simulink model "tests_and_trash"  (R2021b)
settings: Solver=VariableStepAuto  StartTime=0.0  StopTime=TMax  FixedStep=dtMax  MaxStep=dtMax  RelTol=1e-5
undefined symbols (not defined in the file or in its folder): airgap, intensity, pod
libraries: shared6dof x1
settings Model: Creator=Ferran  LastModifiedBy=Ferran
settings SolverCC: MaxConsecutiveMinStep=3

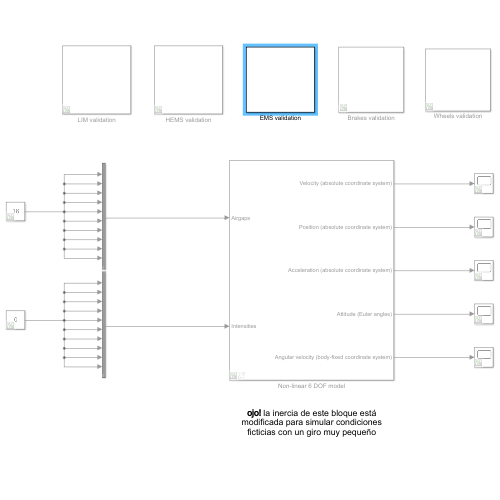
[thumbnail: Simulink's stored preview of the top-level diagram]
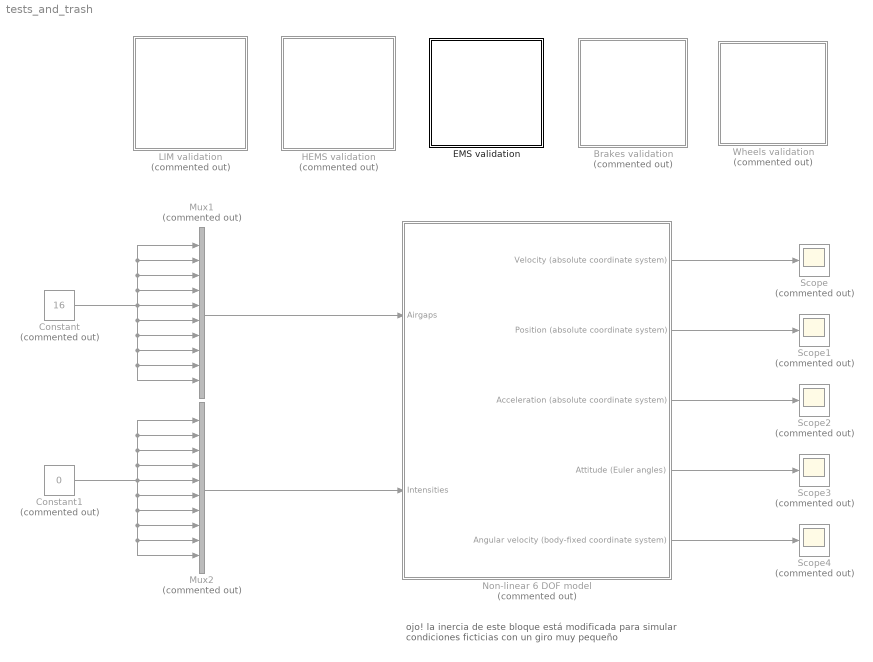
== system tests_and_trash ==
  note: ojo! la inercia de este bloque está modificada para simular condiciones ficticias con un giro muy pequeño
  Brakes validation : Subsystem  Commented=on
  Constant : Constant  Commented=on  Value=16
  Constant1 : Constant  Commented=on  Value=0
  EMS validation : Subsystem
  HEMS validation : Subsystem  Commented=on
  LIM validation : Subsystem  Commented=on
  Mux1 : Mux  Commented=on  Inputs=10
  Mux2 : Mux  Commented=on  Inputs=10
  Non-linear 6 DOF model : Subsystem  Commented=on  AncestorBlock=libH7/Non-linear 6 DOF model
  Scope{,1..4} (5 alike) : Scope  Commented=on
  Wheels validation : Subsystem  Commented=on
  wires:
  Mux2/1 -> Non-linear 6 DOF model/2(Intensities)
  Constant1/1 -> Mux2/2, Mux2/1, Mux2/3, Mux2/4, Mux2/9, Mux2/10, Mux2/8, Mux2/7, Mux2/6, Mux2/5
  Mux1/1 -> Non-linear 6 DOF model/1(Airgaps)
  Non-linear 6 DOF model/1(Velocity (absolute coordinate system)) -> Scope/1
  Non-linear 6 DOF model/2(Position (absolute coordinate system)) -> Scope1/1
  Non-linear 6 DOF model/3(Acceleration (absolute coordinate system)) -> Scope2/1
  Non-linear 6 DOF model/4(Attitude (Euler angles)) -> Scope3/1
  Non-linear 6 DOF model/5(Angular velocity (body-fixed coordinate system)) -> Scope4/1
  Constant/1 -> Mux1/2, Mux1/1, Mux1/3, Mux1/4, Mux1/9, Mux1/10, Mux1/8, Mux1/7, Mux1/6, Mux1/5

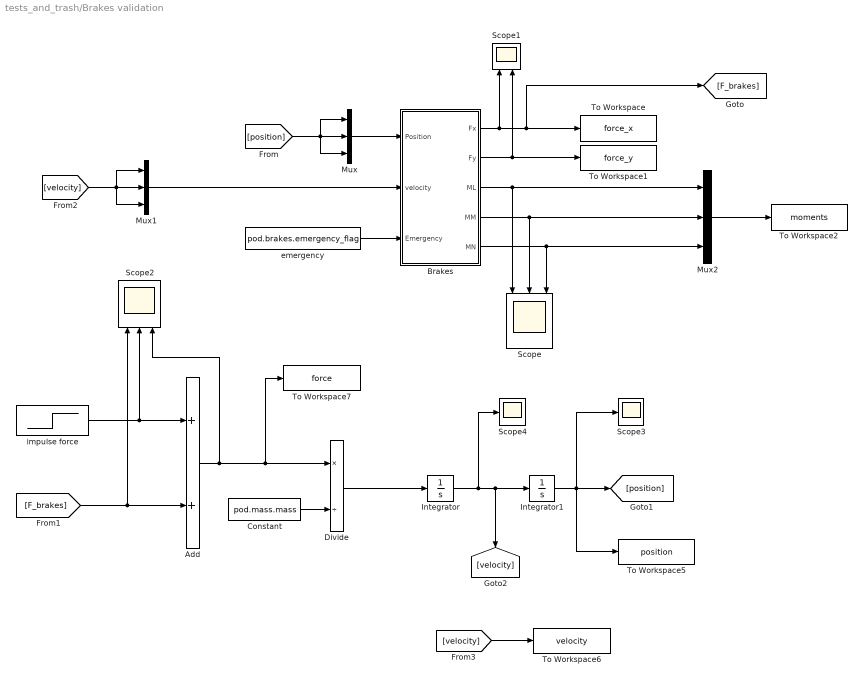
== system tests_and_trash/Brakes validation ==
  Add : Sum  Inputs=2
  Brakes : Subsystem
  Constant : Constant  Value=pod.mass.mass
  Divide : Product  Inputs=*/
  Integrator : Integrator
  Integrator1 : Integrator
  Mux : Mux  Inputs=3
  Mux1 : Mux  Inputs=3
  Mux2 : Mux  Inputs=3
  Scope : Scope  NumInputPorts=3
  Scope1 : Scope  NumInputPorts=2
  Scope2 : Scope  NumInputPorts=3
  Scope3 : Scope
  Scope4 : Scope
  To Workspace : ToWorkspace  VariableName=force_x  SaveFormat=Timeseries  SampleTime=-1
  To Workspace1 : ToWorkspace  VariableName=force_y  SaveFormat=Timeseries  SampleTime=-1
  To Workspace2 : ToWorkspace  VariableName=moments  SaveFormat=Timeseries  SampleTime=-1
  To Workspace5 : ToWorkspace  VariableName=position  SaveFormat=Timeseries  SampleTime=-1
  To Workspace6 : ToWorkspace  VariableName=velocity  SaveFormat=Timeseries  SampleTime=-1
  To Workspace7 : ToWorkspace  VariableName=force  SaveFormat=Timeseries  SampleTime=-1
  emergency : Constant  Value=pod.brakes.emergency_flag
  impulse force : Step  Before=1000  After=0  SampleTime=0
  wires:
  Brakes/1(Fx) -> Scope1/1, To Workspace/1, [F_brakes]
  Brakes/3(ML) -> Scope/1, Mux2/1
  Brakes/2(Fy) -> Scope1/2, To Workspace1/1
  Brakes/5(MN) -> Mux2/3, Scope/3
  emergency/1 -> Brakes/3(Emergency)
  Brakes/4(MM) -> Scope/2, Mux2/2
  impulse force/1 -> Add/1, Scope2/2
  Integrator/1 -> Scope4/1, Integrator1/1, [velocity]
  [F_brakes] -> Add/2, Scope2/1
  Add/1 -> To Workspace7/1, Divide/1, Scope2/3
  Constant/1 -> Divide/2
  Divide/1 -> Integrator/1
  Integrator1/1 -> To Workspace5/1, Scope3/1, [position]
  [position] -> Mux/3, Mux/1, Mux/2
  Mux/1 -> Brakes/1(Position)
  Mux1/1 -> Brakes/2(velocity)
  [velocity] -> Mux1/3, Mux1/1, Mux1/2
  [velocity] -> To Workspace6/1
  Mux2/1 -> To Workspace2/1

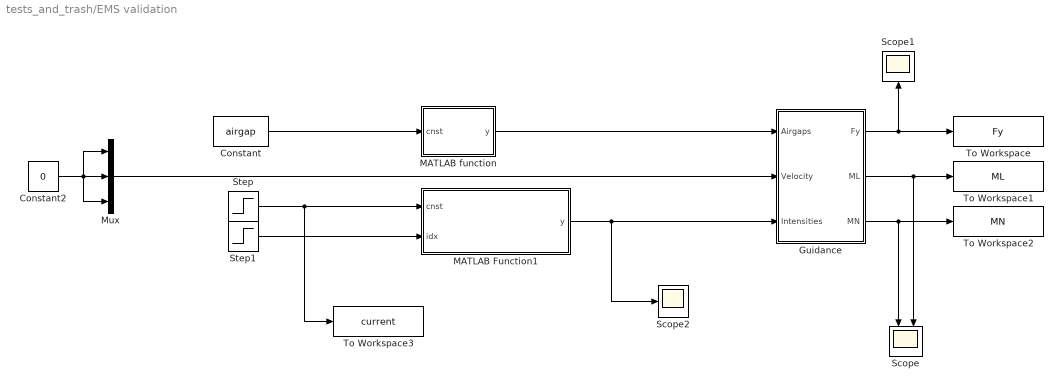
== system tests_and_trash/EMS validation ==
  Constant : Constant  Value=airgap
  Constant2 : Constant  Value=0
  Guidance : Subsystem
  MATLAB Function1 : MATLAB Function  TreatAsAtomicUnit=on
  MATLAB function : MATLAB Function  TreatAsAtomicUnit=on
  Mux : Mux  Inputs=3
  Scope : Scope  NumInputPorts=2
  Scope1 : Scope
  Scope2 : Scope
  Step : Step  Time=3  Before=intensity  After=intensity + 10  SampleTime=0
  Step1 : Step  Time=10  Before=7  After=7  SampleTime=0
  To Workspace : ToWorkspace  VariableName=Fy  SaveFormat=Timeseries  SampleTime=-1
  To Workspace1 : ToWorkspace  VariableName=ML  SaveFormat=Timeseries  SampleTime=-1
  To Workspace2 : ToWorkspace  VariableName=MN  SaveFormat=Timeseries  SampleTime=-1
  To Workspace3 : ToWorkspace  VariableName=current  SaveFormat=Timeseries  SampleTime=-1
  wires:
  Mux/1 -> Guidance/2(Velocity)
  Step/1 -> To Workspace3/1, MATLAB Function1/1(cnst)
  MATLAB function/1(y) -> Guidance/1(Airgaps)
  Constant/1 -> MATLAB function/1(cnst)
  Constant2/1 -> Mux/2, Mux/1, Mux/3
  Step1/1 -> MATLAB Function1/2(idx)
  Guidance/1(Fy) -> To Workspace/1, Scope1/1
  MATLAB Function1/1(y) -> Scope2/1, Guidance/3(Intensities)
  Guidance/2(ML) -> Scope/2, To Workspace1/1
  Guidance/3(MN) -> Scope/1, To Workspace2/1

== system tests_and_trash/HEMS validation ==
  Constant : Constant  Value=airgap
  Constant1 : Constant  Value=intensity
  Constant2 : Constant  Value=5
  Levitation : Subsystem
  MATLAB Function1 : MATLAB Function  TreatAsAtomicUnit=on
  MATLAB unction3 : MATLAB Function  TreatAsAtomicUnit=on
  Mux : Mux  Inputs=3
  Scope : Scope  NumInputPorts=2
  Scope1 : Scope  NumInputPorts=2
  Scope2 : Scope
  To Workspace : ToWorkspace  VariableName=Fx  SaveFormat=Timeseries  SampleTime=-1
  To Workspace1 : ToWorkspace  VariableName=Fz  SaveFormat=Timeseries  SampleTime=-1
  To Workspace2 : ToWorkspace  VariableName=ML  SaveFormat=Timeseries  SampleTime=-1
  To Workspace3 : ToWorkspace  VariableName=MM  SaveFormat=Timeseries  SampleTime=-1
  wires:
  Constant/1 -> MATLAB unction3/1(cnst)
  MATLAB unction3/1(y) -> Levitation/1(Airgaps)
  Constant1/1 -> MATLAB Function1/1(cnst)
  MATLAB Function1/1(y) -> Scope2/1, Levitation/3(Intensities)
  Mux/1 -> Levitation/2(Velocity)
  Levitation/1(Fx) -> Scope/2, To Workspace/1
  Levitation/2(Fz) -> Scope/1, To Workspace1/1
  Levitation/3(ML) -> To Workspace2/1, Scope1/2
  Levitation/4(MM) -> Scope1/1, To Workspace3/1
  Constant2/1 -> Mux/2, Mux/1, Mux/3

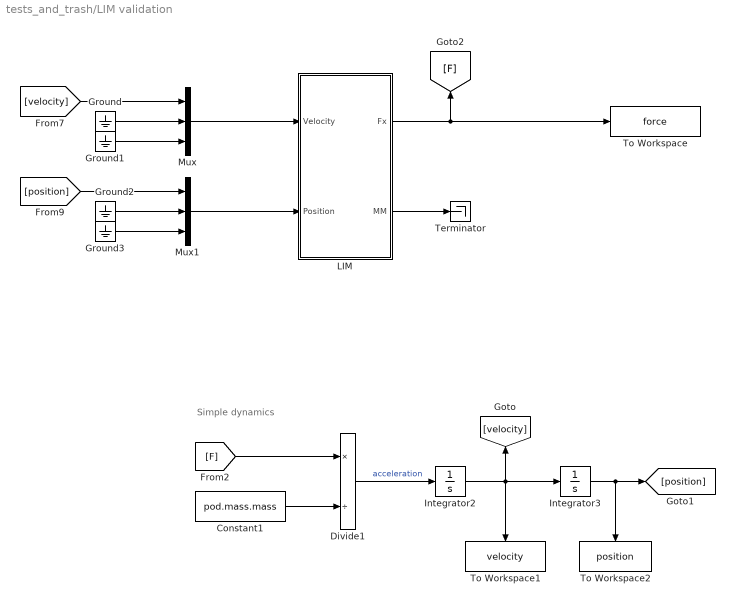
== system tests_and_trash/LIM validation ==
  note: Simple dynamics
  Constant1 : Constant  Value=pod.mass.mass
  Divide1 : Product  Inputs=*/
  Ground{,1..3} (4 alike) : Ground
  Integrator2 : Integrator
  Integrator3 : Integrator
  LIM : Subsystem
  Mux : Mux  Inputs=3
  Mux1 : Mux  Inputs=3
  Terminator : Terminator
  To Workspace : ToWorkspace  VariableName=force  SaveFormat=Timeseries  SampleTime=-1
  To Workspace1 : ToWorkspace  VariableName=velocity  SaveFormat=Timeseries  SampleTime=-1
  To Workspace2 : ToWorkspace  VariableName=position  SaveFormat=Timeseries  SampleTime=-1
  wires:
  Ground/1 -> Mux/2
  Mux/1 -> LIM/1(Velocity)
  Mux1/1 -> LIM/2(Position)
  Ground3/1 -> Mux1/3
  Ground1/1 -> Mux/3
  [velocity] -> Mux/1
  Ground2/1 -> Mux1/2
  [position] -> Mux1/1
  LIM/2(MM) -> Terminator/1
  LIM/1(Fx) -> To Workspace/1, [F]
  [F] -> Divide1/1
  Constant1/1 -> Divide1/2
  Divide1/1 -> Integrator2/1  "acceleration"
  Integrator2/1 -> To Workspace1/1, [velocity], Integrator3/1
  Integrator3/1 -> [position], To Workspace2/1

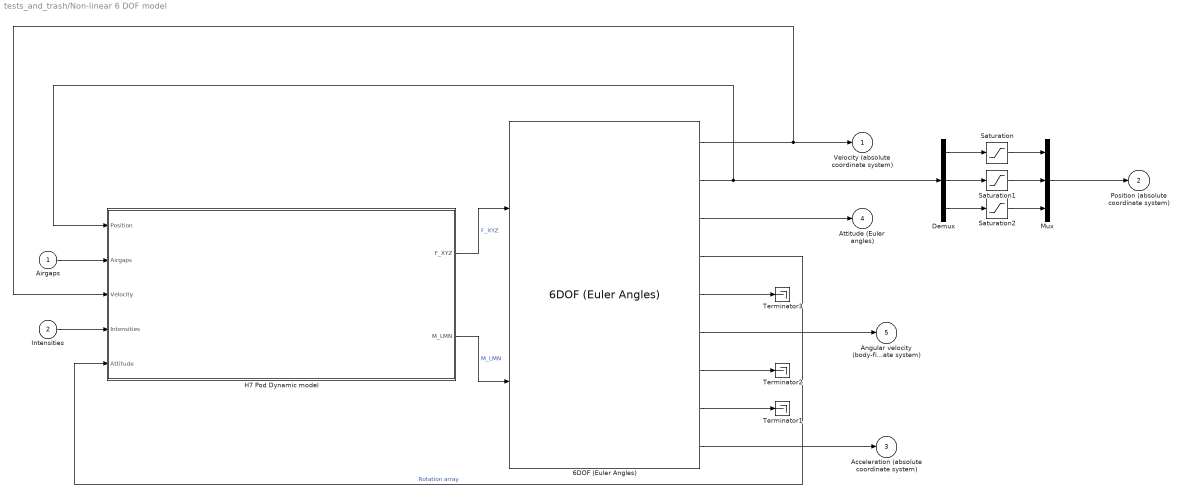
== system tests_and_trash/Non-linear 6 DOF model ==
  Airgaps : Inport
  Intensities : Inport  Port=2
  6DOF (Euler Angles) : shared6dof/6DOF (Euler Angles)  units=Metric (MKS)  mtype=Fixed  rep=Euler Angles  xme_0=initial_conds.x_0  Vm_0=initial_conds.v_0  eul_0=initial_conds.ang_0  pm_0=initial_conds.w_0  mass_0=pod.mass.mass  mass_e=0.5  mass_f=2.0  inertia=pod.mass.inertia * 1e6  inertia_e=eye(3)  inertia_f=2*eye(3)  k_quat=1.0  vre_flag=on  abi_flag=on  aMode=0  xme_statename=''  Vm_statename=''  eul_statename=''  quat_statename=''  pm_statename=''  mass_statename=''
      link override Abi: Port=9
      settings: SourceProductBaseCode=AE,PW,DR,MT,UV,VE
  Demux : Demux  Outputs=3
  H7 Pod Dynamic model : Subsystem  AncestorBlock=libH7/H7 Pod Dynamic model
      mask Display: image('FBD.png', [0.12 0.12 0.78 0.78]); % Use "Edit Image" on toolstrip to change.
  Mux : Mux  Inputs=3
  Saturation : Saturate  UpperLimit=20  LowerLimit=0
  Saturation1 : Saturate  UpperLimit=0.002  LowerLimit=-0.002
  Saturation2 : Saturate  UpperLimit=0  LowerLimit=-0.011
  Terminator1 : Terminator
  Terminator2 : Terminator
  Terminator3 : Terminator
  Velocity (absolute coordinate system) : Outport
  Position (absolute coordinate system) : Outport  Port=2
  Acceleration (absolute coordinate system) : Outport  Port=3
  Attitude (Euler angles) : Outport  Port=4
  Angular velocity (body-fixed coordinate system) : Outport  Port=5
  wires:
  Mux/1 -> Position (absolute coordinate system)/1
  Saturation2/1 -> Mux/3
  Saturation1/1 -> Mux/2
  Saturation/1 -> Mux/1
  Demux/3 -> Saturation2/1
  Demux/2 -> Saturation1/1
  Demux/1 -> Saturation/1
  Airgaps/1 -> H7 Pod Dynamic model/2(Airgaps)
  6DOF (Euler Angles)/7 -> Terminator2/1
  6DOF (Euler Angles)/5 -> Terminator3/1
  6DOF (Euler Angles)/3 -> Attitude (Euler angles)/1
  6DOF (Euler Angles)/9 -> Acceleration (absolute coordinate system)/1
  6DOF (Euler Angles)/6 -> Angular velocity (body-fixed coordinate system)/1
  6DOF (Euler Angles)/8 -> Terminator1/1
  H7 Pod Dynamic model/2(M_LMN) -> 6DOF (Euler Angles)/2  "M_LMN"
  H7 Pod Dynamic model/1(F_XYZ) -> 6DOF (Euler Angles)/1  "F_XYZ"
  6DOF (Euler Angles)/4 -> H7 Pod Dynamic model/5(Attitude)  "Rotation array"
  Intensities/1 -> H7 Pod Dynamic model/4(Intensities)
  6DOF (Euler Angles)/1 -> H7 Pod Dynamic model/3(Velocity), Velocity (absolute coordinate system)/1
  6DOF (Euler Angles)/2 -> H7 Pod Dynamic model/1(Position), Demux/1

== system tests_and_trash/Wheels validation ==
  Add : Sum
  Mux : Mux  Inputs=3
  Scope : Scope
  Scope1 : Scope
  Scope2 : Scope
  Step : Step  After=5  SampleTime=0
  Step1 : Step  Time=2  After=pod.general.z_range - 5  SampleTime=0
  To Workspace : ToWorkspace  VariableName=z  SaveFormat=Timeseries  SampleTime=-1
  To Workspace1 : ToWorkspace  VariableName=F_x  SaveFormat=Timeseries  SampleTime=-1
  To Workspace2 : ToWorkspace  VariableName=MM  SaveFormat=Timeseries  SampleTime=-1
  Wheels : Subsystem
  wires:
  Wheels/2(MM) -> To Workspace2/1, Scope1/1
  Wheels/1(Fx) -> To Workspace1/1, Scope/1
  Step1/1 -> Add/2
  Step/1 -> Add/1
  Add/1 -> Scope2/1, [z]
  Mux/1 -> Wheels/1(Position)
  [z] -> To Workspace/1, Mux/3, Mux/1, Mux/2

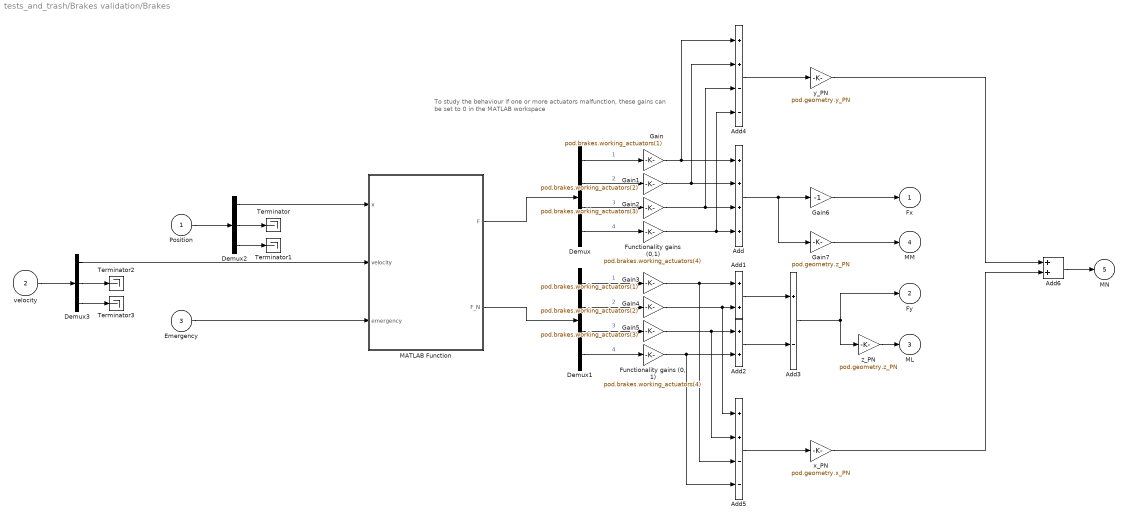
== system tests_and_trash/Brakes validation/Brakes ==
  note: To study the behaviour if one or more actuators malfunction,
      | these gains can be set to 0 in the MATLAB workspace
  Position : Inport
  velocity : Inport  Port=2
  Emergency : Inport  Port=3
  Add : Sum  Inputs=++++
  Add1 : Sum
  Add2 : Sum
  Add3 : Sum  Inputs=+-
  Add4 : Sum  Inputs=++--
  Add5 : Sum  Inputs=++--
  Add6 : Sum
  Demux : Demux
  Demux1 : Demux
  Demux2 : Demux  Outputs=3
  Demux3 : Demux  Outputs=3
  "Functionality gains (0, 1)" : Gain  Gain=pod.brakes.working_actuators(4)
  Functionality gains (0,1) : Gain  Gain=pod.brakes.working_actuators(4)
  Gain : Gain  Gain=pod.brakes.working_actuators(1)
  Gain1 : Gain  Gain=pod.brakes.working_actuators(2)
  Gain2 : Gain  Gain=pod.brakes.working_actuators(3)
  Gain3 : Gain  Gain=pod.brakes.working_actuators(1)
  Gain4 : Gain  Gain=pod.brakes.working_actuators(2)
  Gain5 : Gain  Gain=pod.brakes.working_actuators(3)
  Gain6 : Gain  Gain=-1
  Gain7 : Gain  Gain=pod.geometry.z_PN
  MATLAB Function : MATLAB Function  TreatAsAtomicUnit=on
  Terminator{,1..3} (4 alike) : Terminator
  x_PN : Gain  Gain=pod.geometry.x_PN
  y_PN : Gain  Gain=pod.geometry.y_PN
  z_PN : Gain  Gain=pod.geometry.z_PN
  Fx : Outport
  Fy : Outport  Port=2
  ML : Outport  Port=3
  MM : Outport  Port=4
  MN : Outport  Port=5
  wires:
  Emergency/1 -> MATLAB Function/3(emergency)
  MATLAB Function/1(F) -> Demux/1
  Demux/1 -> Gain/1  "1"
  Demux/2 -> Gain1/1  "2"
  Demux/3 -> Gain2/1  "3"
  Demux/4 -> Functionality gains (0,1)/1  "4"
  Demux1/4 -> "Functionality gains (0, 1)"/1  "4"
  Demux1/3 -> Gain5/1  "3"
  Demux1/1 -> Gain3/1  "1"
  Demux1/2 -> Gain4/1  "2"
  MATLAB Function/2(F_N) -> Demux1/1
  Functionality gains (0,1)/1 -> Add4/4, Add/4
  Gain2/1 -> Add4/3, Add/3
  Gain1/1 -> Add4/2, Add/2
  Gain/1 -> Add4/1, Add/1
  Add/1 -> Gain7/1, Gain6/1
  Gain6/1 -> Fx/1
  Gain4/1 -> Add5/1, Add1/2
  Gain3/1 -> Add1/1, Add5/3
  Gain5/1 -> Add5/2, Add2/1
  "Functionality gains (0, 1)"/1 -> Add2/2, Add5/4
  Add1/1 -> Add3/1
  Add2/1 -> Add3/2
  Add3/1 -> z_PN/1, Fy/1
  z_PN/1 -> ML/1
  Gain7/1 -> MM/1
  Add4/1 -> y_PN/1
  Demux2/3 -> Terminator1/1
  Position/1 -> Demux2/1
  Demux2/1 -> MATLAB Function/1(x)
  Demux2/2 -> Terminator/1
  velocity/1 -> Demux3/1
  Demux3/2 -> Terminator2/1
  Demux3/3 -> Terminator3/1
  Demux3/1 -> MATLAB Function/2(velocity)
  Add5/1 -> x_PN/1
  Add6/1 -> MN/1
  y_PN/1 -> Add6/1
  x_PN/1 -> Add6/2

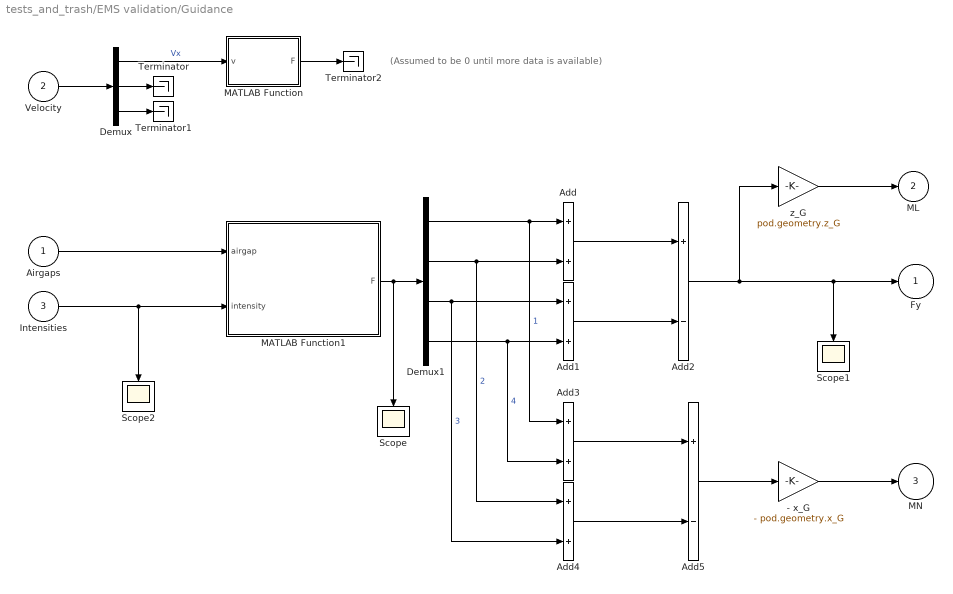
== system tests_and_trash/EMS validation/Guidance ==
  note: (Assumed to be 0 until more data is available)
  Airgaps : Inport
  Velocity : Inport  Port=2
  Intensities : Inport  Port=3
  - x_G : Gain  Gain=- pod.geometry.x_G
  Add{,1,3..4} (4 alike) : Sum
  Add2 : Sum  Inputs=+-
  Add5 : Sum  Inputs=+-
  Demux : Demux  Outputs=3
  Demux1 : Demux
  MATLAB Function : MATLAB Function  TreatAsAtomicUnit=on
  MATLAB Function1 : MATLAB Function  TreatAsAtomicUnit=on
  Scope : Scope
  Scope1 : Scope
  Scope2 : Scope
  Terminator : Terminator
  Terminator1 : Terminator
  Terminator2 : Terminator
  z_G : Gain  Gain=pod.geometry.z_G
  Fy : Outport
  ML : Outport  Port=2
  MN : Outport  Port=3
  wires:
  Demux/1 -> MATLAB Function/1(v)  "Vx"
  Velocity/1 -> Demux/1
  Demux/2 -> Terminator/1
  Demux/3 -> Terminator1/1
  MATLAB Function/1(F) -> Terminator2/1
  MATLAB Function1/1(F) -> Demux1/1, Scope/1
  Intensities/1 -> Scope2/1, MATLAB Function1/2(intensity)
  Airgaps/1 -> MATLAB Function1/1(airgap)
  Demux1/1 -> Add3/1, Add/1  "1"
  Demux1/2 -> Add4/1, Add/2  "2"
  Demux1/3 -> Add4/2, Add1/1  "3"
  Demux1/4 -> Add3/2, Add1/2  "4"
  Add1/1 -> Add2/2
  Add/1 -> Add2/1
  Add2/1 -> z_G/1, Scope1/1, Fy/1
  z_G/1 -> ML/1
  Add3/1 -> Add5/1
  Add4/1 -> Add5/2
  Add5/1 -> - x_G/1
  - x_G/1 -> MN/1

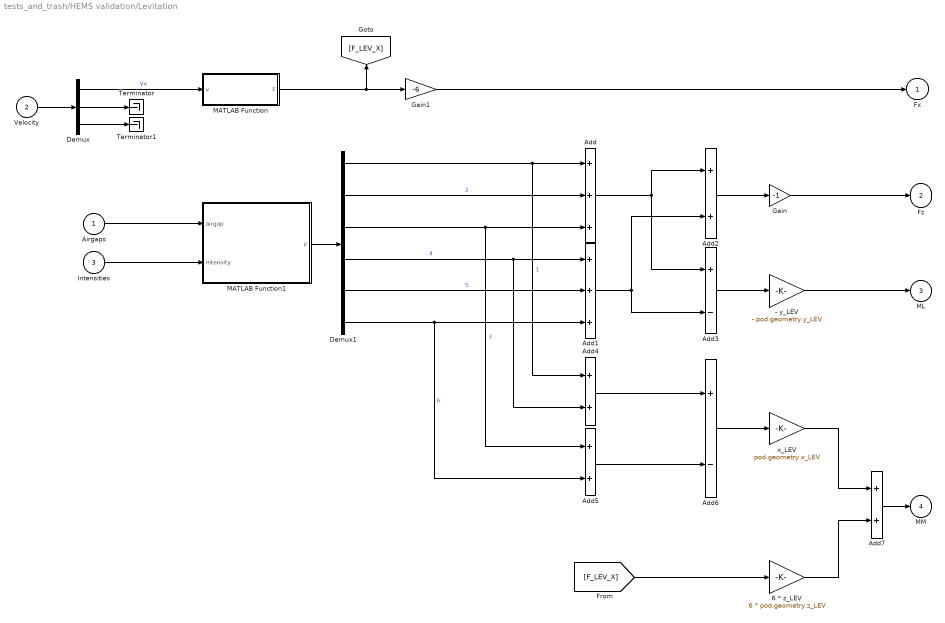
== system tests_and_trash/HEMS validation/Levitation ==
  Airgaps : Inport
  Velocity : Inport  Port=2
  Intensities : Inport  Port=3
  - y_LEV : Gain  Gain=- pod.geometry.y_LEV
  6 * z_LEV : Gain  Gain=6 * pod.geometry.z_LEV
  Add : Sum  Inputs=+++
  Add1 : Sum  Inputs=+++
  Add{2,4..5,7} (4 alike) : Sum
  Add3 : Sum  Inputs=+-
  Add6 : Sum  Inputs=+-
  Demux : Demux  Outputs=3
  Demux1 : Demux  Outputs=6
  Gain : Gain  Gain=-1
  Gain1 : Gain  Gain=-6
  MATLAB Function : MATLAB Function  TreatAsAtomicUnit=on
  MATLAB Function1 : MATLAB Function  TreatAsAtomicUnit=on
  Terminator : Terminator
  Terminator1 : Terminator
  x_LEV : Gain  Gain=pod.geometry.x_LEV
  Fx : Outport
  Fz : Outport  Port=2
  ML : Outport  Port=3
  MM : Outport  Port=4
  wires:
  Demux/2 -> Terminator/1
  Demux/3 -> Terminator1/1
  Velocity/1 -> Demux/1
  Demux/1 -> MATLAB Function/1(v)  "Vx"
  Airgaps/1 -> MATLAB Function1/1(airgap)
  Intensities/1 -> MATLAB Function1/2(intensity)
  MATLAB Function1/1(F) -> Demux1/1
  Gain/1 -> Fz/1
  Demux1/1 -> Add4/1, Add/1  "1"
  Demux1/2 -> Add/2  "2"
  Demux1/3 -> Add5/1, Add/3  "3"
  Demux1/4 -> Add4/2, Add1/1  "4"
  Demux1/5 -> Add1/2  "5"
  Demux1/6 -> Add5/2, Add1/3  "6"
  Add/1 -> Add2/1, Add3/1
  Add1/1 -> Add2/2, Add3/2
  Add2/1 -> Gain/1
  Add3/1 -> - y_LEV/1
  - y_LEV/1 -> ML/1
  Gain1/1 -> Fx/1
  [F_LEV_X] -> 6 * z_LEV/1
  Add4/1 -> Add6/1
  Add5/1 -> Add6/2
  Add6/1 -> x_LEV/1
  Add7/1 -> MM/1
  x_LEV/1 -> Add7/1
  6 * z_LEV/1 -> Add7/2
  MATLAB Function/1(F) -> [F_LEV_X], Gain1/1

== system tests_and_trash/LIM validation/LIM ==
  note: Note that it is assumed that the transversal forces are compensated
  Velocity : Inport
  Position : Inport  Port=2
  Demux : Demux  Outputs=3
  Demux1 : Demux  Outputs=3
  MATLAB Function : MATLAB Function  TreatAsAtomicUnit=on
  MATLAB Function1 : MATLAB Function  TreatAsAtomicUnit=on
  Product : Product
  Terminator{,1..3} (4 alike) : Terminator
  z_LIM : Gain  Gain=pod.geometry.z_LIM
  Fx : Outport
  MM : Outport  Port=2
  wires:
  Velocity/1 -> Demux/1
  Demux/2 -> Terminator/1
  Demux/3 -> Terminator1/1
  Demux/1 -> MATLAB Function1/1(v), MATLAB Function/1(v)  "Vx"
  Position/1 -> Demux1/1
  Demux1/3 -> Terminator3/1
  Demux1/2 -> Terminator2/1
  Demux1/1 -> MATLAB Function1/2(x)  "X"
  MATLAB Function1/1(sign) -> Product/2
  MATLAB Function/1(F) -> Product/1
  Product/1 -> z_LIM/1, Fx/1
  z_LIM/1 -> MM/1

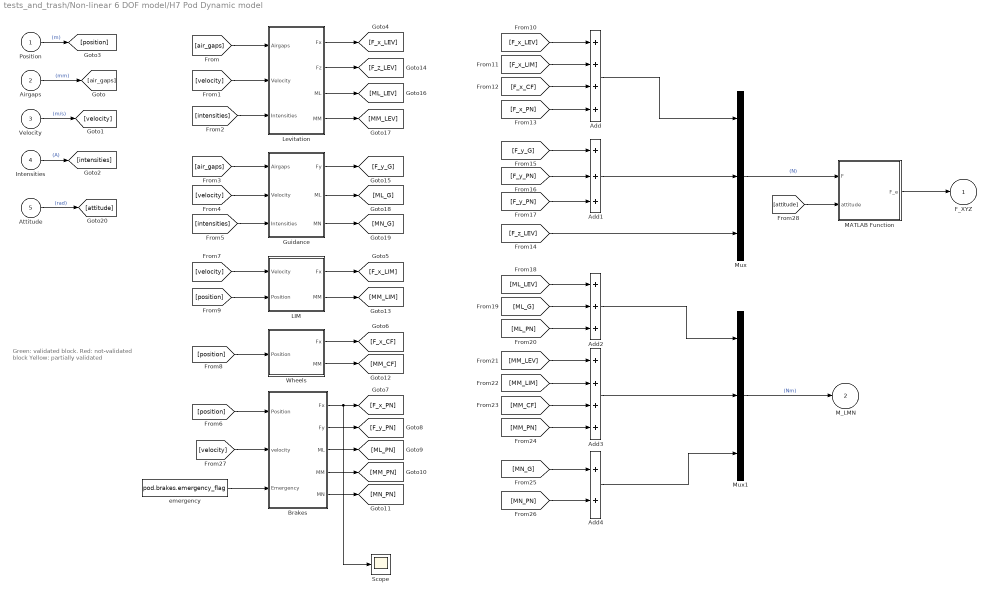
== system tests_and_trash/Non-linear 6 DOF model/H7 Pod Dynamic model ==
  note: Green: validated block.
      | Red: not-validated block
      | Yellow: partially validated
  Position : Inport
  Airgaps : Inport  Port=2
  Velocity : Inport  Port=3
  Intensities : Inport  Port=4
  Attitude : Inport  Port=5
  Add : Sum  Inputs=++++
  Add1 : Sum  Inputs=+++
  Add2 : Sum  Inputs=+++
  Add3 : Sum  Inputs=++++
  Add4 : Sum
  Brakes : Subsystem
  Guidance : Subsystem
  LIM : Subsystem
  Levitation : Subsystem
  MATLAB Function : MATLAB Function  TreatAsAtomicUnit=on
  Mux : Mux  Inputs=3
  Mux1 : Mux  Inputs=3
  Scope : Scope
  Wheels : Subsystem
  emergency : Constant  Value=pod.brakes.emergency_flag
  F_XYZ : Outport
  M_LMN : Outport  Port=2
  wires:
  MATLAB Function/1(F_e) -> F_XYZ/1
  [attitude] -> MATLAB Function/2(attitude)
  Attitude/1 -> [attitude]  "(rad)"
  [velocity] -> Brakes/2(velocity)
  Add4/1 -> Mux1/3
  [MN_G] -> Add4/1
  [MN_PN] -> Add4/2
  [MM_CF] -> Add3/3
  [MM_LIM] -> Add3/2
  Add3/1 -> Mux1/2
  [MM_PN] -> Add3/4
  [MM_LEV] -> Add3/1
  [ML_PN] -> Add2/3
  [ML_G] -> Add2/2
  Add2/1 -> Mux1/1
  [ML_LEV] -> Add2/1
  Add1/1 -> Mux/2
  [F_y_PN] -> Add1/3
  [F_y_PN] -> Add1/2
  [F_y_G] -> Add1/1
  [F_z_LEV] -> Mux/3
  [F_x_PN] -> Add/4
  [F_x_CF] -> Add/3
  [F_x_LIM] -> Add/2
  [F_x_LEV] -> Add/1
  Add/1 -> Mux/1
  Guidance/3(MN) -> [MN_G]
  Guidance/2(ML) -> [ML_G]
  Levitation/4(MM) -> [MM_LEV]
  Levitation/3(ML) -> [ML_LEV]
  Guidance/1(Fy) -> [F_y_G]
  Levitation/2(Fz) -> [F_z_LEV]
  LIM/2(MM) -> [MM_LIM]
  Wheels/2(MM) -> [MM_CF]
  Brakes/5(MN) -> [MN_PN]
  Brakes/4(MM) -> [MM_PN]
  Brakes/3(ML) -> [ML_PN]
  Brakes/2(Fy) -> [F_y_PN]
  Brakes/1(Fx) -> Scope/1, [F_x_PN]
  Wheels/1(Fx) -> [F_x_CF]
  LIM/1(Fx) -> [F_x_LIM]
  Levitation/1(Fx) -> [F_x_LEV]
  [position] -> LIM/2(Position)
  [position] -> Wheels/1(Position)
  emergency/1 -> Brakes/3(Emergency)
  [position] -> Brakes/1(Position)
  Position/1 -> [position]  "(m)"
  [velocity] -> LIM/1(Velocity)
  [air_gaps] -> Guidance/1(Airgaps)
  [intensities] -> Guidance/3(Intensities)
  [velocity] -> Guidance/2(Velocity)
  [intensities] -> Levitation/3(Intensities)
  [velocity] -> Levitation/2(Velocity)
  [air_gaps] -> Levitation/1(Airgaps)
  Mux1/1 -> M_LMN/1  "(Nm)"
  Mux/1 -> MATLAB Function/1(F)  "(N)"
  Intensities/1 -> [intensities]  "(A)"
  Velocity/1 -> [velocity]  "(m/s)"
  Airgaps/1 -> [air_gaps]  "(mm)"

== system tests_and_trash/Wheels validation/Wheels ==
  Position : Inport
  Demux : Demux  Outputs=3
  MATLAB Function : MATLAB Function  TreatAsAtomicUnit=on
  Product : Product
  Terminator : Terminator
  Terminator1 : Terminator
  Fx : Outport
  MM : Outport  Port=2
  wires:
  Position/1 -> Demux/1
  Demux/2 -> Terminator/1
  Demux/3 -> MATLAB Function/1(z)
  MATLAB Function/1(F) -> Fx/1, Product/1
  Demux/1 -> Terminator1/1
  MATLAB Function/2(z_CF) -> Product/2
  Product/1 -> MM/1

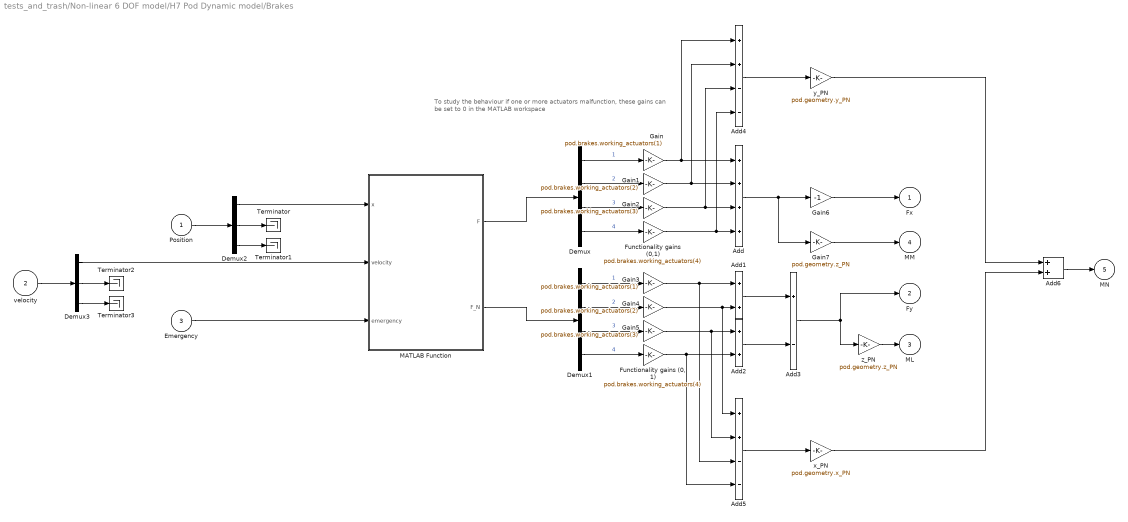
== system tests_and_trash/Non-linear 6 DOF model/H7 Pod Dynamic model/Brakes ==
  note: To study the behaviour if one or more actuators malfunction,
      | these gains can be set to 0 in the MATLAB workspace
  Position : Inport
  velocity : Inport  Port=2
  Emergency : Inport  Port=3
  Add : Sum  Inputs=++++
  Add1 : Sum
  Add2 : Sum
  Add3 : Sum  Inputs=+-
  Add4 : Sum  Inputs=++--
  Add5 : Sum  Inputs=++--
  Add6 : Sum
  Demux : Demux
  Demux1 : Demux
  Demux2 : Demux  Outputs=3
  Demux3 : Demux  Outputs=3
  "Functionality gains (0, 1)" : Gain  Gain=pod.brakes.working_actuators(4)
  Functionality gains (0,1) : Gain  Gain=pod.brakes.working_actuators(4)
  Gain : Gain  Gain=pod.brakes.working_actuators(1)
  Gain1 : Gain  Gain=pod.brakes.working_actuators(2)
  Gain2 : Gain  Gain=pod.brakes.working_actuators(3)
  Gain3 : Gain  Gain=pod.brakes.working_actuators(1)
  Gain4 : Gain  Gain=pod.brakes.working_actuators(2)
  Gain5 : Gain  Gain=pod.brakes.working_actuators(3)
  Gain6 : Gain  Gain=-1
  Gain7 : Gain  Gain=pod.geometry.z_PN
  MATLAB Function : MATLAB Function  TreatAsAtomicUnit=on
  Terminator{,1..3} (4 alike) : Terminator
  x_PN : Gain  Gain=pod.geometry.x_PN
  y_PN : Gain  Gain=pod.geometry.y_PN
  z_PN : Gain  Gain=pod.geometry.z_PN
  Fx : Outport
  Fy : Outport  Port=2
  ML : Outport  Port=3
  MM : Outport  Port=4
  MN : Outport  Port=5
  wires:
  x_PN/1 -> Add6/2
  y_PN/1 -> Add6/1
  Add6/1 -> MN/1
  Add5/1 -> x_PN/1
  Demux3/1 -> MATLAB Function/2(velocity)
  Demux3/3 -> Terminator3/1
  Demux3/2 -> Terminator2/1
  velocity/1 -> Demux3/1
  Demux2/2 -> Terminator/1
  Demux2/1 -> MATLAB Function/1(x)
  Position/1 -> Demux2/1
  Demux2/3 -> Terminator1/1
  Add4/1 -> y_PN/1
  Gain7/1 -> MM/1
  z_PN/1 -> ML/1
  Add3/1 -> Fy/1, z_PN/1
  Add2/1 -> Add3/2
  Add1/1 -> Add3/1
  "Functionality gains (0, 1)"/1 -> Add5/4, Add2/2
  Gain5/1 -> Add2/1, Add5/2
  Gain3/1 -> Add5/3, Add1/1
  Gain4/1 -> Add1/2, Add5/1
  Gain6/1 -> Fx/1
  Add/1 -> Gain6/1, Gain7/1
  Gain/1 -> Add/1, Add4/1
  Gain1/1 -> Add/2, Add4/2
  Gain2/1 -> Add/3, Add4/3
  Functionality gains (0,1)/1 -> Add/4, Add4/4
  MATLAB Function/2(F_N) -> Demux1/1
  Demux1/2 -> Gain4/1  "2"
  Demux1/1 -> Gain3/1  "1"
  Demux1/3 -> Gain5/1  "3"
  Demux1/4 -> "Functionality gains (0, 1)"/1  "4"
  Demux/4 -> Functionality gains (0,1)/1  "4"
  Demux/3 -> Gain2/1  "3"
  Demux/2 -> Gain1/1  "2"
  Demux/1 -> Gain/1  "1"
  MATLAB Function/1(F) -> Demux/1
  Emergency/1 -> MATLAB Function/3(emergency)

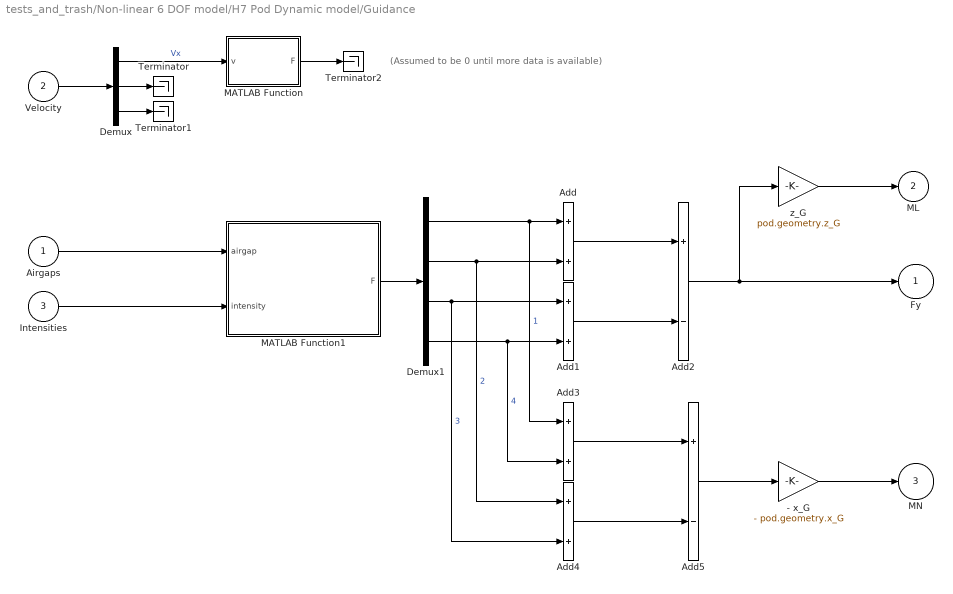
== system tests_and_trash/Non-linear 6 DOF model/H7 Pod Dynamic model/Guidance ==
  note: (Assumed to be 0 until more data is available)
  Airgaps : Inport
  Velocity : Inport  Port=2
  Intensities : Inport  Port=3
  - x_G : Gain  Gain=- pod.geometry.x_G
  Add{,1,3..4} (4 alike) : Sum
  Add2 : Sum  Inputs=+-
  Add5 : Sum  Inputs=+-
  Demux : Demux  Outputs=3
  Demux1 : Demux
  MATLAB Function : MATLAB Function  TreatAsAtomicUnit=on
  MATLAB Function1 : MATLAB Function  TreatAsAtomicUnit=on
  Terminator : Terminator
  Terminator1 : Terminator
  Terminator2 : Terminator
  z_G : Gain  Gain=pod.geometry.z_G
  Fy : Outport
  ML : Outport  Port=2
  MN : Outport  Port=3
  wires:
  - x_G/1 -> MN/1
  Add5/1 -> - x_G/1
  Add4/1 -> Add5/2
  Add3/1 -> Add5/1
  z_G/1 -> ML/1
  Add2/1 -> Fy/1, z_G/1
  Add/1 -> Add2/1
  Add1/1 -> Add2/2
  Demux1/4 -> Add1/2, Add3/2  "4"
  Demux1/3 -> Add1/1, Add4/2  "3"
  Demux1/2 -> Add/2, Add4/1  "2"
  Demux1/1 -> Add/1, Add3/1  "1"
  Airgaps/1 -> MATLAB Function1/1(airgap)
  Intensities/1 -> MATLAB Function1/2(intensity)
  MATLAB Function1/1(F) -> Demux1/1
  MATLAB Function/1(F) -> Terminator2/1
  Demux/3 -> Terminator1/1
  Demux/2 -> Terminator/1
  Velocity/1 -> Demux/1
  Demux/1 -> MATLAB Function/1(v)  "Vx"

== system tests_and_trash/Non-linear 6 DOF model/H7 Pod Dynamic model/LIM ==
  note: Note that it is assumed that the transversal forces are compensated
  Velocity : Inport
  Position : Inport  Port=2
  Demux : Demux  Outputs=3
  Demux1 : Demux  Outputs=3
  MATLAB Function : MATLAB Function  TreatAsAtomicUnit=on
  MATLAB Function1 : MATLAB Function  TreatAsAtomicUnit=on
  Product : Product
  Terminator{,1..3} (4 alike) : Terminator
  z_LIM : Gain  Gain=pod.geometry.z_LIM
  Fx : Outport
  MM : Outport  Port=2
  wires:
  z_LIM/1 -> MM/1
  Product/1 -> Fx/1, z_LIM/1
  MATLAB Function/1(F) -> Product/1
  MATLAB Function1/1(sign) -> Product/2
  Demux1/1 -> MATLAB Function1/2(x)  "X"
  Demux1/2 -> Terminator2/1
  Demux1/3 -> Terminator3/1
  Position/1 -> Demux1/1
  Demux/1 -> MATLAB Function/1(v), MATLAB Function1/1(v)  "Vx"
  Demux/3 -> Terminator1/1
  Demux/2 -> Terminator/1
  Velocity/1 -> Demux/1

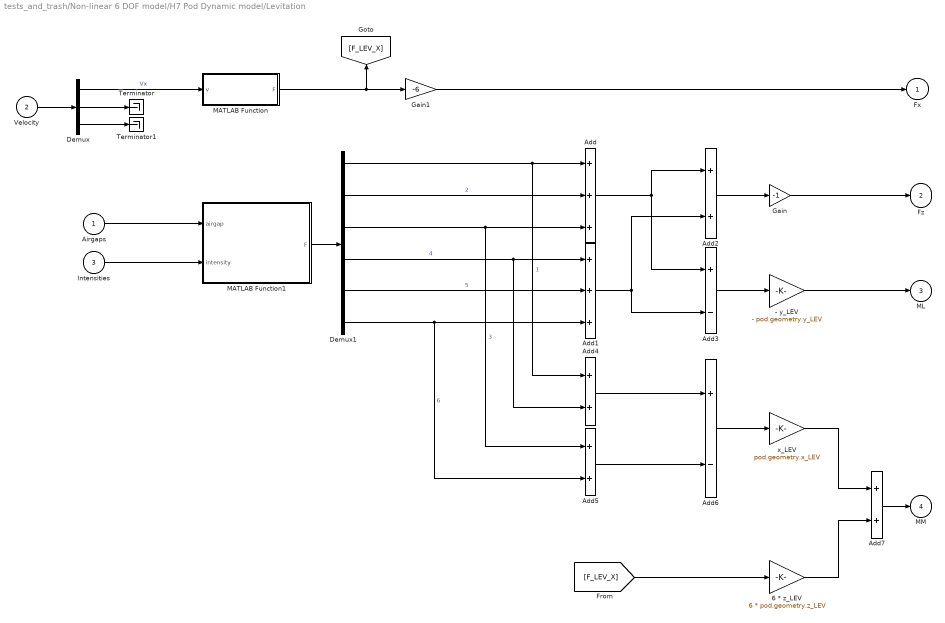
== system tests_and_trash/Non-linear 6 DOF model/H7 Pod Dynamic model/Levitation ==
  Airgaps : Inport
  Velocity : Inport  Port=2
  Intensities : Inport  Port=3
  - y_LEV : Gain  Gain=- pod.geometry.y_LEV
  6 * z_LEV : Gain  Gain=6 * pod.geometry.z_LEV
  Add : Sum  Inputs=+++
  Add1 : Sum  Inputs=+++
  Add{2,4..5,7} (4 alike) : Sum
  Add3 : Sum  Inputs=+-
  Add6 : Sum  Inputs=+-
  Demux : Demux  Outputs=3
  Demux1 : Demux  Outputs=6
  Gain : Gain  Gain=-1
  Gain1 : Gain  Gain=-6
  MATLAB Function : MATLAB Function  TreatAsAtomicUnit=on
  MATLAB Function1 : MATLAB Function  TreatAsAtomicUnit=on
  Terminator : Terminator
  Terminator1 : Terminator
  x_LEV : Gain  Gain=pod.geometry.x_LEV
  Fx : Outport
  Fz : Outport  Port=2
  ML : Outport  Port=3
  MM : Outport  Port=4
  wires:
  MATLAB Function/1(F) -> Gain1/1, [F_LEV_X]
  6 * z_LEV/1 -> Add7/2
  x_LEV/1 -> Add7/1
  Add7/1 -> MM/1
  Add6/1 -> x_LEV/1
  Add5/1 -> Add6/2
  Add4/1 -> Add6/1
  [F_LEV_X] -> 6 * z_LEV/1
  Gain1/1 -> Fx/1
  - y_LEV/1 -> ML/1
  Add3/1 -> - y_LEV/1
  Add2/1 -> Gain/1
  Add1/1 -> Add3/2, Add2/2
  Add/1 -> Add3/1, Add2/1
  Demux1/6 -> Add1/3, Add5/2  "6"
  Demux1/5 -> Add1/2  "5"
  Demux1/4 -> Add1/1, Add4/2  "4"
  Demux1/3 -> Add/3, Add5/1  "3"
  Demux1/2 -> Add/2  "2"
  Demux1/1 -> Add/1, Add4/1  "1"
  Gain/1 -> Fz/1
  MATLAB Function1/1(F) -> Demux1/1
  Intensities/1 -> MATLAB Function1/2(intensity)
  Airgaps/1 -> MATLAB Function1/1(airgap)
  Demux/1 -> MATLAB Function/1(v)  "Vx"
  Velocity/1 -> Demux/1
  Demux/3 -> Terminator1/1
  Demux/2 -> Terminator/1

== system tests_and_trash/Non-linear 6 DOF model/H7 Pod Dynamic model/Wheels ==
  Position : Inport
  Demux : Demux  Outputs=3
  MATLAB Function : MATLAB Function  TreatAsAtomicUnit=on
  Product : Product
  Terminator : Terminator
  Terminator1 : Terminator
  Fx : Outport
  MM : Outport  Port=2
  wires:
  Product/1 -> MM/1
  MATLAB Function/2(z_CF) -> Product/2
  Demux/1 -> Terminator1/1
  MATLAB Function/1(F) -> Product/1, Fx/1
  Demux/3 -> MATLAB Function/1(z)
  Demux/2 -> Terminator/1
  Position/1 -> Demux/1

== matlab function tests_and_trash/Wheels validation/Wheels/MATLAB Function ==
  data: z input; F output; pod parameter; z_CF output
function [F, z_CF] = rollingFriction(z, pod)
% Computes the rolling resistance force (N) of the wheels. It distinguishes
% 3 cases: 
%   (1) z = 0. Pod touching the ground
%   (2) z = z_max. Pod touching the ceiling. It is assumed no current
%   applied to the HEMS. 
%   (3) Otherwise. Pod levitating. 
% ═════════════════════════════════════════════════════════════════════════
% Last updated: 20.12.2021
% ═════════════════════════════════════════════════════════════════════════

% F_LEV worst case scenario computation
x   = 12; % [mm]
y   = 0;  % [A]

F_LEV = pod.levitation.poly_1_unit.p00 + ...
        pod.levitation.poly_1_unit.p10.*x + ...
        pod.levitation.poly_1_unit.p01.*y + ...
        pod.levitation.poly_1_unit.p20.*x.^2 + ...
        pod.levitation.poly_1_unit.p11.*x.*y + ...
        pod.levitation.poly_1_unit.p02.*y.^2 + ...
        pod.levitation.poly_1_unit.p21.*x.^2.*y + ...
        pod.levitation.poly_1_unit.p12.*x.*y.^2 + ...
        pod.levitation.poly_1_unit.p03.*y.^3;

% Main algorithm
if z == 0
    F_N   = pod.mass.mass * 9.81;
    z_CF  = - pod.geometry.z_CF;
elseif z == pod.general.z_range
    F_N   = 6 * F_LEV - pod.mass.mass * 9.81;
    z_CF  = pod.geometry.z_CF;
else
    F_N   = 0;
    z_CF  = 0;
end

F = pod.wheels.number * pod.wheels.roll_coef * F_N;

== matlab function tests_and_trash/Non-linear 6 DOF model/H7 Pod Dynamic model/Brakes/MATLAB Function ==
  data: x input; velocity input; F output; emergency input; F_N output; pod parameter
function [F, F_N] = brakes_activation(x, velocity, emergency, pod)
% Computes the braking force of the pneumatic actuators if and only if 
%     (1) The emergency flag has been raised
%     (2) The pod is above the acceleration phase distance
% ═════════════════════════════════════════════════════════════════════════
% Last updated: 20.12.2021
% ═════════════════════════════════════════════════════════════════════════

if (emergency == 1 && x >= pod.brakes.d && velocity >= 0)
    F       = pod.brakes.force * ones(pod.brakes.n,1);
    F_N     = pod.brakes.normal_force * ones(pod.brakes.n,1);
else
    F       = zeros(pod.brakes.n,1);
    F_N     = zeros(pod.brakes.n,1);
end

== matlab function tests_and_trash/HEMS validation/Levitation/MATLAB Function ==
  data: v input; F output; pod parameter
function F = HEMSdrag(v, pod)
% Computes the drag force (N) of one HEMS unit as a function of the 
% velocity (m/s)
% ═════════════════════════════════════════════════════════════════════════
% Last updated: 15.12.2021
% ═════════════════════════════════════════════════════════════════════════

F = pod.levitation.drag_1_unit.poly.p3*v^3 + ...
    pod.levitation.drag_1_unit.poly.p2*v^2 + ...
    pod.levitation.drag_1_unit.poly.p1*v   + ...
    pod.levitation.drag_1_unit.poly.p0;

== matlab function tests_and_trash/Non-linear 6 DOF model/H7 Pod Dynamic model/Guidance/MATLAB Function ==
  data: v input; F output
function F = EMSdrag(v)
% Computes the drag force (N) of one EMS units as a function of 
% its velocity (m/s)
% ═════════════════════════════════════════════════════════════════════════
% Last updated: 15.12.2021
% ════════════════════════════════════════════════════════════════════════

F = 0;

== matlab function tests_and_trash/Non-linear 6 DOF model/H7 Pod Dynamic model/Guidance/MATLAB Function1 ==
  data: airgap input; F output; intensity input; pod parameter
function F = EMSlev(airgap, intensity, pod)
% Computes the levitation force (N) of all the EMS units as a function of 
% their air gaps (mm) and intensities (A)
% ═════════════════════════════════════════════════════════════════════════
% Last updated: 15.12.2021
% ════════════════════════════════════════════════════════════════════════

x   = airgap(7:10);
y   = intensity(7:10);

F = pod.guiding.poly.p00 + ...
    pod.guiding.poly.p10.*x + ...
    pod.guiding.poly.p01.*y + ...
    pod.guiding.poly.p20.*x.^2 + ...
    pod.guiding.poly.p11.*x.*y + ...
    pod.guiding.poly.p02.*y.^2 + ...
    pod.guiding.poly.p21.*x.^2.*y + ...
    pod.guiding.poly.p12.*x.*y.^2 + ...
    pod.guiding.poly.p03.*y.^3;

== matlab function tests_and_trash/Non-linear 6 DOF model/H7 Pod Dynamic model/LIM/MATLAB Function ==
  data: v input; F output; pod parameter
function F = LIMtraction(v, pod)
% Computes the traction force (N) of the LIM as a function of 
% the absolute velocity of the prototype (m/s)
% ═════════════════════════════════════════════════════════════════════════
% Last updated: 20.12.2021
% ═════════════════════════════════════════════════════════════════════════

F = pod.propulsion.poly.p3*v^3 + ...
    pod.propulsion.poly.p2*v^2 + ...
    pod.propulsion.poly.p1*v   + ...
    pod.propulsion.poly.p0;

== matlab function tests_and_trash/Non-linear 6 DOF model/H7 Pod Dynamic model/LIM/MATLAB Function1 ==
  data: v input; x input; sign output; pod parameter
function sign = LIMdirection(v, x, pod)
% Decides if the LIM force is being applied to accelerate or to brake 
% by comparing the position of the pod with a predefined treshold
% ═════════════════════════════════════════════════════════════════════════
% Last updated: 20.12.2021
% ═════════════════════════════════════════════════════════════════════════

if x >= pod.brakes.d && v > 0    
    sign = -1;
elseif x >= pod.brakes.d && v <= 0
    sign = 0;
else
    sign = 1;
end

== matlab function tests_and_trash/Non-linear 6 DOF model/H7 Pod Dynamic model/Levitation/MATLAB Function ==
  data: v input; F output; pod parameter
function F = HEMSdrag(v, pod)
% Computes the drag force (N) of one HEMS unit as a function of the 
% velocity (m/s)
% ═════════════════════════════════════════════════════════════════════════
% Last updated: 15.12.2021
% ═════════════════════════════════════════════════════════════════════════

F = pod.levitation.drag_1_unit.poly.p3*v^3 + ...
    pod.levitation.drag_1_unit.poly.p2*v^2 + ...
    pod.levitation.drag_1_unit.poly.p1*v   + ...
    pod.levitation.drag_1_unit.poly.p0;

== matlab function tests_and_trash/Non-linear 6 DOF model/H7 Pod Dynamic model/Levitation/MATLAB Function1 ==
  data: airgap input; F output; intensity input; pod parameter
function F = HEMSlev(airgap, intensity, pod)
% Computes the levitation force (N) of all the HEMS units as a function of 
% their air gaps (mm) and intensities (A)
% ═════════════════════════════════════════════════════════════════════════
% Last updated: 15.12.2021
% ════════════════════════════════════════════════════════════════════════

x   = airgap(1:6);
y   = intensity(1:6);

F = pod.levitation.poly_1_unit.p00 + ...
    pod.levitation.poly_1_unit.p10.*x + ...
    pod.levitation.poly_1_unit.p01.*y + ...
    pod.levitation.poly_1_unit.p20.*x.^2 + ...
    pod.levitation.poly_1_unit.p11.*x.*y + ...
    pod.levitation.poly_1_unit.p02.*y.^2 + ...
    pod.levitation.poly_1_unit.p21.*x.^2.*y + ...
    pod.levitation.poly_1_unit.p12.*x.*y.^2 + ...
    pod.levitation.poly_1_unit.p03.*y.^3;

== matlab function tests_and_trash/Non-linear 6 DOF model/H7 Pod Dynamic model/MATLAB Function ==
  data: F input; F_e output; attitude input; pod parameter
function F_e = BF2E(F, attitude, pod)
% Computes the total force in absoute axis
% ═════════════════════════════════════════════════════════════════════════
% Last updated: 27.12.2021
% ═════════════════════════════════════════════════════════════════════════
F     = reshape(F, [3 1]);


F_e = attitude * F + pod.mass.mass * [0 0 9.81]';

== matlab function tests_and_trash/Non-linear 6 DOF model/H7 Pod Dynamic model/Wheels/MATLAB Function ==
  data: z input; F output; pod parameter; z_CF output
function [F, z_CF] = rollingFriction(z, pod)
% Computes the rolling resistance force (N) of the wheels. It distinguishes
% 3 cases: 
%   (1) z = 0. Pod touching the ground
%   (2) z = z_max. Pod touching the ceiling. It is assumed no current
%   applied to the HEMS. 
%   (3) Otherwise. Pod levitating. 
% ═════════════════════════════════════════════════════════════════════════
% Last updated: 26.12.2021
% ═════════════════════════════════════════════════════════════════════════

% F_LEV worst case scenario computation
x   = 12; % [mm]
y   = 0;  % [A]

F_LEV = pod.levitation.poly_1_unit.p00 + ...
        pod.levitation.poly_1_unit.p10.*x + ...
        pod.levitation.poly_1_unit.p01.*y + ...
        pod.levitation.poly_1_unit.p20.*x.^2 + ...
        pod.levitation.poly_1_unit.p11.*x.*y + ...
        pod.levitation.poly_1_unit.p02.*y.^2 + ...
        pod.levitation.poly_1_unit.p21.*x.^2.*y + ...
        pod.levitation.poly_1_unit.p12.*x.*y.^2 + ...
        pod.levitation.poly_1_unit.p03.*y.^3;

% Main algorithm
if z == 0
    F_N   = pod.mass.mass * 9.81;
    z_CF  = - pod.geometry.z_CF;
elseif z == pod.general.z_range
    F_N   = 6 * F_LEV - pod.mass.mass * 9.81;
    z_CF  = pod.geometry.z_CF;
else
    F_N   = 0;
    z_CF  = 0;
end

F = pod.wheels.number * pod.wheels.roll_coef * F_N;

== matlab function tests_and_trash/EMS validation/Guidance/MATLAB Function ==
  data: v input; F output
function F = EMSdrag(v)
% Computes the drag force (N) of one EMS units as a function of 
% its velocity (m/s)
% ═════════════════════════════════════════════════════════════════════════
% Last updated: 15.12.2021
% ════════════════════════════════════════════════════════════════════════

F = 0;

== matlab function tests_and_trash/HEMS validation/Levitation/MATLAB Function1 ==
  data: airgap input; F output; intensity input; pod parameter
function F = HEMSlev(airgap, intensity, pod)
% Computes the levitation force (N) of all the HEMS units as a function of 
% their air gaps (mm) and intensities (A)
% ═════════════════════════════════════════════════════════════════════════
% Last updated: 15.12.2021
% ════════════════════════════════════════════════════════════════════════

x   = airgap(1:6);
y   = intensity(1:6);

F = pod.levitation.poly_1_unit.p00 + ...
    pod.levitation.poly_1_unit.p10.*x + ...
    pod.levitation.poly_1_unit.p01.*y + ...
    pod.levitation.poly_1_unit.p20.*x.^2 + ...
    pod.levitation.poly_1_unit.p11.*x.*y + ...
    pod.levitation.poly_1_unit.p02.*y.^2 + ...
    pod.levitation.poly_1_unit.p21.*x.^2.*y + ...
    pod.levitation.poly_1_unit.p12.*x.*y.^2 + ...
    pod.levitation.poly_1_unit.p03.*y.^3;

== matlab function tests_and_trash/HEMS validation/MATLAB Function1 ==
  data: y output; cnst input
function y = vectorizer_changer(cnst)



y = cnst * ones(10,1);

== matlab function tests_and_trash/EMS validation/Guidance/MATLAB Function1 ==
  data: airgap input; F output; intensity input; pod parameter
function F = EMSlev(airgap, intensity, pod)
% Computes the levitation force (N) of all the EMS units as a function of 
% their air gaps (mm) and intensities (A)
% ═════════════════════════════════════════════════════════════════════════
% Last updated: 15.12.2021
% ════════════════════════════════════════════════════════════════════════

x   = airgap(7:10);
y   = intensity(7:10);

F = pod.guiding.poly.p00 + ...
    pod.guiding.poly.p10.*x + ...
    pod.guiding.poly.p01.*y + ...
    pod.guiding.poly.p20.*x.^2 + ...
    pod.guiding.poly.p11.*x.*y + ...
    pod.guiding.poly.p02.*y.^2 + ...
    pod.guiding.poly.p21.*x.^2.*y + ...
    pod.guiding.poly.p12.*x.*y.^2 + ...
    pod.guiding.poly.p03.*y.^3;

== matlab function tests_and_trash/LIM validation/LIM/MATLAB Function ==
  data: v input; F output; pod parameter
function F = LIMtraction(v, pod)
% Computes the traction force (N) of the LIM as a function of 
% the absolute velocity of the prototype (m/s)
% ═════════════════════════════════════════════════════════════════════════
% Last updated: 20.12.2021
% ═════════════════════════════════════════════════════════════════════════

F = pod.propulsion.poly.p3*v^3 + ...
    pod.propulsion.poly.p2*v^2 + ...
    pod.propulsion.poly.p1*v   + ...
    pod.propulsion.poly.p0;

== matlab function tests_and_trash/LIM validation/LIM/MATLAB Function1 ==
  data: v input; x input; sign output; pod parameter
function sign = LIMdirection(v, x, pod)
% Decides if the LIM force is being applied to accelerate or to brake 
% by comparing the position of the pod with a predefined treshold
% ═════════════════════════════════════════════════════════════════════════
% Last updated: 20.12.2021
% ═════════════════════════════════════════════════════════════════════════

if x >= pod.brakes.d && v > 0    
    sign = -1;

elseif x >= pod.brakes.d && v <= 0
    sign = 0;

else
    sign = 1;
end

== matlab function tests_and_trash/HEMS validation/MATLAB unction3 ==
  data: y output; cnst input
function y = vectorizer(cnst)

y = cnst * ones(10,1);

== matlab function tests_and_trash/EMS validation/MATLAB Function1 ==
  data: y output; cnst input; idx input
function y = vectorizer_changer(cnst, idx)



y = zeros(10,1);
y(idx) = cnst;

== matlab function tests_and_trash/EMS validation/MATLAB function ==
  data: y output; cnst input
function y = vectorizer(cnst)

y = cnst * ones(10,1);

== matlab function tests_and_trash/Brakes validation/Brakes/MATLAB Function ==
  data: x input; velocity input; F output; emergency input; F_N output; pod parameter
function [F, F_N] = brakes_activation(x, velocity, emergency, pod)
% Computes the braking force of the pneumatic actuators if and only if 
%     (1) The emergency flag has been raised
%     (2) The pod is above the acceleration phase distance
% ═════════════════════════════════════════════════════════════════════════
% Last updated: 20.12.2021
% ═════════════════════════════════════════════════════════════════════════

if (emergency == 1 && x >= pod.brakes.d && velocity >= 0)
    F       = pod.brakes.force * ones(pod.brakes.n,1);
    F_N     = pod.brakes.normal_force * ones(pod.brakes.n,1);
else
    F       = zeros(pod.brakes.n,1);
    F_N     = zeros(pod.brakes.n,1);
end
